simulink model "Copy_of_planar1R_2R"  (R2022b)
settings: Solver=VariableStepAuto  StartTime=0.0  StopTime=100  FixedStep=0.001  RelTol=1e-6
model workspace (MAT data in the model file):
  LC = Simulink.Signal
  LC.DataType = 'double'
  LC.Dimensions = 1
  LC.DimensionsMode = 'auto'
  LC.Complexity = 'real'
  LC.SampleTime = -1
  LC.SamplingMode = 'auto'
  LC.InitialValue = '1'
  fsA = Simulink.Signal
  fsA.DataType = 'double'
  fsA.Dimensions = 1
  fsA.DimensionsMode = 'auto'
  fsA.Complexity = 'real'
  fsA.SampleTime = -1
  fsA.SamplingMode = 'auto'
  fsA.InitialValue = '0.0'
  fsC = Simulink.Signal
  fsC.DataType = 'double'
  fsC.Dimensions = 1
  fsC.DimensionsMode = 'auto'
  fsC.Complexity = 'real'
  fsC.SampleTime = -1
  fsC.SamplingMode = 'auto'
  fsC.InitialValue = '0'
  fvA = Simulink.Signal
  fvA.DataType = 'double'
  fvA.Dimensions = 1
  fvA.DimensionsMode = 'auto'
  fvA.Complexity = 'real'
  fvA.SampleTime = -1
  fvA.SamplingMode = 'auto'
  fvA.InitialValue = '0.0'
  fvC = Simulink.Signal
  fvC.DataType = 'double'
  fvC.Dimensions = 1
  fvC.DimensionsMode = 'auto'
  fvC.Complexity = 'real'
  fvC.SampleTime = -1
  fvC.SamplingMode = 'auto'
  fvC.InitialValue = '0.0'
  g0 = Simulink.Signal
  g0.DataType = 'double'
  g0.Dimensions = 1
  g0.DimensionsMode = 'auto'
  g0.Complexity = 'real'
  g0.SampleTime = -1
  g0.SamplingMode = 'auto'
  g0.InitialValue = '9.8'
  iAxx = Simulink.Signal
  iAxx.DataType = 'double'
  iAxx.Dimensions = 1
  iAxx.DimensionsMode = 'auto'
  iAxx.Complexity = 'real'
  iAxx.SampleTime = -1
  iAxx.SamplingMode = 'auto'
  iAxx.InitialValue = '0.0'
  iCxx = Simulink.Signal
  iCxx.DataType = 'double'
  iCxx.Dimensions = 1
  iCxx.DimensionsMode = 'auto'
  iCxx.Complexity = 'real'
  iCxx.SampleTime = -1
  iCxx.SamplingMode = 'auto'
  iCxx.InitialValue = '0'
  lA = Simulink.Signal
  lA.DataType = 'double'
  lA.Dimensions = 1
  lA.DimensionsMode = 'auto'
  lA.Complexity = 'real'
  lA.SampleTime = -1
  lA.SamplingMode = 'auto'
  lA.InitialValue = '0.54'
  lC = Simulink.Signal
  lC.DataType = 'double'
  lC.Dimensions = 1
  lC.DimensionsMode = 'auto'
  lC.Complexity = 'real'
  lC.SampleTime = -1
  lC.SamplingMode = 'auto'
  lC.InitialValue = '1'
  mA = Simulink.Signal
  mA.DataType = 'double'
  mA.Dimensions = 1
  mA.DimensionsMode = 'auto'
  mA.Complexity = 'real'
  mA.SampleTime = -1
  mA.SamplingMode = 'auto'
  mA.InitialValue = '1'
  mC = Simulink.Signal
  mC.DataType = 'double'
  mC.Dimensions = 1
  mC.DimensionsMode = 'auto'
  mC.Complexity = 'real'
  mC.SampleTime = -1
  mC.SamplingMode = 'auto'
  mC.InitialValue = '1'
settings Model: Creator=giancarlo  LastModifiedBy=giancarlo

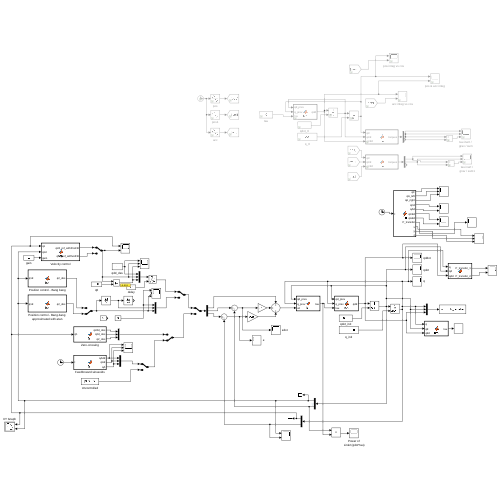
[thumbnail: Simulink's stored preview of the top-level diagram]
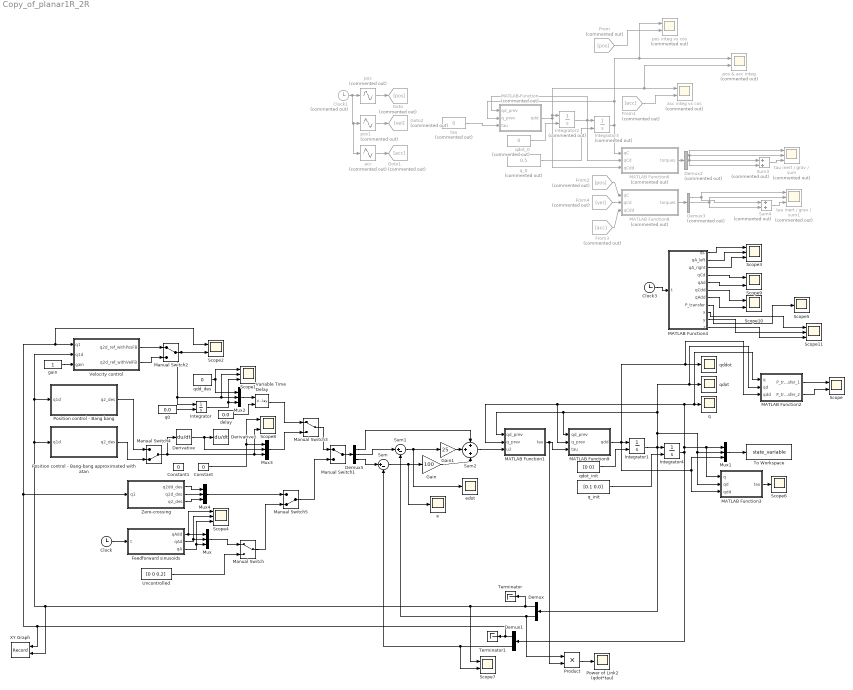
== system Copy_of_planar1R_2R ==
  Clock : Clock
  Clock1 : Clock  Commented=on
  Clock3 : Clock
  Constant : Constant  Value=0
  Constant1 : Constant  Value=0
  Demux : Demux  Outputs=2
  Demux1 : Demux  Outputs=2
  Demux2 : Demux  Commented=on  Outputs=[1 1 2 ]
  Demux3 : Demux  Commented=on  Outputs=[1 1 2 ]
  Demux5 : Demux  Outputs=3
  Derivative : Derivative
  Derivative1 : Derivative
  Feedforward sinusoids : MATLAB Function  TreatAsAtomicUnit=on
  From : From  Commented=on  GotoTag=pos
  From1 : From  Commented=on  GotoTag=acc
  From2 : From  Commented=on  GotoTag=pos
  From3 : From  Commented=on  GotoTag=acc
  From4 : From  Commented=on  GotoTag=vel
  Gain : Gain  Gain=100
  Gain1 : Gain  Gain=25
  Goto : Goto  Commented=on  GotoTag=pos
  Goto1 : Goto  Commented=on  GotoTag=acc
  Goto2 : Goto  Commented=on  GotoTag=vel
  Integrator : Integrator  InitialConditionSource=external  InitialCondition=0.3
  Integrator1 : Integrator  InitialConditionSource=external  InitialCondition=[0 0]
  Integrator2 : Integrator  Commented=on  InitialConditionSource=external  InitialCondition=[0 0]
  Integrator3 : Integrator  Commented=on  InitialConditionSource=external  InitialCondition=[0 0]
  Integrator4 : Integrator  InitialConditionSource=external  InitialCondition=[0 0]
  MATLAB Function : MATLAB Function  Commented=on  TreatAsAtomicUnit=on
  MATLAB Function1 : MATLAB Function  TreatAsAtomicUnit=on
  MATLAB Function2 : MATLAB Function  TreatAsAtomicUnit=on
  MATLAB Function3 : MATLAB Function  TreatAsAtomicUnit=on
  MATLAB Function4 : MATLAB Function  TreatAsAtomicUnit=on
  MATLAB Function6 : MATLAB Function  Commented=on  TreatAsAtomicUnit=on
  MATLAB Function8 : MATLAB Function  Commented=on  TreatAsAtomicUnit=on
  MATLAB Function9 : MATLAB Function  TreatAsAtomicUnit=on
  Manual Switch{,1..3} (4 alike) : ManualSwitch
  Manual Switch4 : ManualSwitch  CurrentSetting=0
  Manual Switch5 : ManualSwitch  CurrentSetting=0
  Mux{,1..4} (5 alike) : Mux  Inputs=3
  Position control - Bang bang : MATLAB Function  TreatAsAtomicUnit=on
  Position control - Bang-bang approximated with atan : MATLAB Function  TreatAsAtomicUnit=on
  Power of Link2 (qdot*tau) : Scope
  Product : Product
  Scope{,2,7,9..10} (5 alike) : Scope  NumInputPorts=2
  Scope{1,3..4,8,11} (5 alike) : Scope  NumInputPorts=3
  Scope5 : Scope
  Scope6 : Scope
  Sum : Sum  Inputs=|+-
  Sum1 : Sum  Inputs=|+-
  Sum2 : Sum  Inputs=+++
  Sum3 : Sum  Commented=on
  Sum4 : Sum  Commented=on
  Terminator : Terminator
  Terminator1 : Terminator
  To Workspace : ToWorkspace  VariableName=state_variable  SaveFormat=Timeseries  SampleTime=-1
  Uncontrolled : Constant  Value=[0 0 0.2]
  Variable Time Delay : VariableTransportDelay  MaximumDelay=10
  Velocity control : MATLAB Function  TreatAsAtomicUnit=on
  XY Graph : Record  FileSettingsInternal="{\"entries\":[{\"content\":{\"excelSettings\":{\"content\":{},\"type\":\"Streamout.ExcelSettings\"}},\"type\":\"Streamout.FileSettingStorage\",\"uuid\":\"17f3f7c0-a543-4966-915e-296ee2588332\"}],\"packageUris\":[\"http://schema.mathworks.com/mf0/streamout_blocks/R2020a\"],\"version\":\"1.0\"}"  Layout=[1 1]  SignalsInternal="{\"entries\":[{\"content\":{\"signals\":[{\"content\":{\"blockPath\":[\"Copy_of_planar1R_2R/XY Graph\"],\"channel\":[],\"dimensions\":[1],\"domain\":\"Copy_of_planar1R_2R/XY Graph\",\"lineColor\":\"#a2142f\",\"plots\":[1],\"port\":1,\"sid\":[\"\"],\"signalID\":42397,\"signalName\":\"Demux1:1\"},\"type\":\"RecordBlkView.Signal\",\"uuid\":\"0ab6503b-74ed-4c5b-b113-e67b91689d53\"},{\"content\":{\"blockPath\":[\"Copy_of_planar1R_2R/XY Graph\"],\"channel\":[],\"dimensions\":[1],\"domain\":\"Copy_of_planar1R_2R/XY Graph\",\"lineColor\":\"#139fff\",\"plots\":[1],\"port\":2,\"sid\":[\"\"],\"signalID\":42401,\"signalName\":\"Demux:1\"},\"type\":\"RecordBlkView.Signal\",\"uuid\":\"fae32842-6c35-404d-92af-908aeb941329\"}]},\"type\":\"RecordBlkView.InputSignals\",\"uuid\":\"726fd067-675c-490d-8cf4-42f1baed3ed2\"}],\"packageUris\":[\"http://schema.mathworks.com/mf0/streamout_blocks/R2020a\"],\"version\":\"1.0\"}"  VisualizationBindings="{\"xyplotplugin\":{\"info\":[{\"series\":[{\"bindingParametersList\":[{\"parameter\":\"X-Axis\",\"signalID\":42397,\"signalName\":\"Demux1:1\"},{\"parameter\":\"Y-Axis\",\"signalID\":42401,\"signalName\":\"Demux:1\"}],\"seriesID\":10957}],\"subplotID\":1}]}}"  CompatibilityTag=XY
  Zero-crossing : MATLAB Function  TreatAsAtomicUnit=on
  acc : Sin  Commented=on  TimeSource=Use external signal  Amplitude=-0.5*(2*pi*0.261145458563799)^2  Frequency=2*pi*0.261145458563799  Phase=pi/2  SampleTime=0
  acc integ vs cos : Scope  Commented=on  NumInputPorts=2
  delay : Constant  Value=0.0
  e : Scope
  edot : Scope
  gain : Constant
  pos : Sin  Commented=on  TimeSource=Use external signal  Amplitude=0.5  Frequency=2*pi*(0.261145458563799)  Phase=pi/2  SampleTime=0
  pos & acc integ : Scope  Commented=on  NumInputPorts=2
  pos integ vs cos : Scope  Commented=on  NumInputPorts=2
  pos1 : Sin  Commented=on  TimeSource=Use external signal  Amplitude=0.5*(2*pi*(0.261145458563799))  Frequency=2*pi*(0.261145458563799)  Phase=pi  SampleTime=0
  q : Scope
  q0 : Constant  Value=0.0
  q_0 : Constant  Commented=on  Value=0.5
  q_init : Constant  Value=[0.1 0.0]
  qdd_des : Constant  Value=0
  qddot : Scope
  qdot : Scope
  qdot_0 : Constant  Commented=on  Value=0
  qdot_init : Constant  Value=[0 0]
  tau : Constant  Commented=on  Value=0
  tau inert / grav / sum : Scope  Commented=on  NumInputPorts=3
  tau inert / grav / sum1 : Scope  Commented=on  NumInputPorts=3
  wires:
  qdot_0/1 -> Integrator2/2
  Integrator2/1 -> MATLAB Function6/2(qCd), MATLAB Function/1(qd_prev), Integrator3/1
  MATLAB Function/1(qdd) -> pos & acc integ/2, acc integ vs cos/1, Integrator2/1, MATLAB Function6/3(qCdd)
  q_0/1 -> Integrator3/2
  Integrator3/1 -> MATLAB Function6/1(qC), pos & acc integ/1, pos integ vs cos/1, MATLAB Function/2(q_prev)
  tau/1 -> MATLAB Function/3(tau)
  MATLAB Function6/1(torques) -> Demux2/1
  Demux2/1 -> Sum3/1, tau inert / grav / sum/1
  Demux2/2 -> tau inert / grav / sum/2, Sum3/2
  Sum3/1 -> tau inert / grav / sum/3
  From/1 -> pos integ vs cos/2
  From1/1 -> acc integ vs cos/2
  From2/1 -> MATLAB Function8/1(qC)
  From4/1 -> MATLAB Function8/2(qCd)
  Clock1/1 -> pos1/1, acc/1, pos/1
  pos/1 -> Goto/1
  acc/1 -> Goto1/1
  From3/1 -> MATLAB Function8/3(qCdd)
  pos1/1 -> Goto2/1
  Sum4/1 -> tau inert / grav / sum1/3
  MATLAB Function8/1(torques) -> Demux3/1
  Demux3/2 -> tau inert / grav / sum1/2, Sum4/2
  Demux3/1 -> Sum4/1, tau inert / grav / sum1/1
  Integrator4/1 -> Mux1/1, MATLAB Function3/1(q), MATLAB Function2/1(q), q/1, MATLAB Function1/2(q_prev), MATLAB Function9/2(q_prev), Demux1/1
  Demux/2 -> Sum1/2, Product/1
  Demux1/2 -> Scope7/2, Sum/2
  Gain1/1 -> Sum2/2
  q_init/1 -> Integrator4/2
  Sum/1 -> e/1, Gain/1
  Demux1/1 -> XY Graph/1, Scope2/1, Velocity control/1(q1), Zero-crossing/1(q1), Terminator1/1
  Sum1/1 -> Gain1/1, edot/1
  qdot_init/1 -> Integrator1/2
  MATLAB Function9/1(qdd) -> qddot/1, MATLAB Function2/3(qdd), Integrator1/1, Mux1/3, MATLAB Function3/3(qdd)
  Demux/1 -> Terminator/1, Scope7/1, XY Graph/2, Velocity control/2(q1d), Position control - Bang bang/1(q1d), Position control - Bang-bang approximated with atan/1(q1d)
  Gain/1 -> Sum2/3
  MATLAB Function1/1(tau) -> Product/2, MATLAB Function9/3(tau)
  Sum2/1 -> MATLAB Function1/3(u2)
  Clock/1 -> Feedforward sinusoids/1(t)
  Feedforward sinusoids/1(qAdd) -> Scope4/1, Mux/1
  Feedforward sinusoids/3(qA) -> Mux/3, Scope4/3
  Feedforward sinusoids/2(qAd) -> Scope4/2, Mux/2
  Manual Switch2/1 -> Scope2/2, Scope1/2, Mux2/2, Integrator/1
  q0/1 -> Integrator/2
  Uncontrolled/1 -> Manual Switch/2
  Mux/1 -> Manual Switch/1
  Demux5/1 -> Sum2/1
  Demux5/2 -> Sum1/1
  Demux5/3 -> Sum/1
  Mux1/1 -> To Workspace/1
  Integrator1/1 -> qdot/1, MATLAB Function2/2(qd), MATLAB Function9/1(qd_prev), MATLAB Function1/1(qd_prev), MATLAB Function3/2(qd), Mux1/2, Demux/1, Integrator4/1
  MATLAB Function3/1(tau) -> Scope6/1
  Manual Switch1/1 -> Demux5/1
  Mux2/1 -> Variable Time Delay/1
  Integrator/1 -> Mux2/3, Scope1/3
  qdd_des/1 -> Mux2/1, Scope1/1
  delay/1 -> Variable Time Delay/2
  gain/1 -> Velocity control/3(gain)
  Velocity control/1(q2d_ref_withPosFB) -> Manual Switch2/1
  Velocity control/2(q2d_ref_withVelFB) -> Manual Switch2/2
  Mux3/1 -> Manual Switch3/2
  Variable Time Delay/1 -> Manual Switch3/1
  Manual Switch3/1 -> Manual Switch1/1
  Product/1 -> Power of Link2 (qdot*tau)/1
  Constant/1 -> Scope8/1, Mux3/1
  Position control - Bang-bang approximated with atan/1(q2_des) -> Manual Switch4/2
  Position control - Bang bang/1(q2_des) -> Manual Switch4/1
  Manual Switch4/1 -> Scope8/3, Mux3/3, Derivative/1
  Derivative/1 -> Mux3/2, Derivative1/1
  Zero-crossing/1(q2dd_des) -> Mux4/1
  Zero-crossing/2(q2d_des) -> Mux4/2
  Zero-crossing/3(q2_des) -> Mux4/3
  Manual Switch/1 -> Manual Switch5/2
  Manual Switch5/1 -> Manual Switch1/2
  Mux4/1 -> Manual Switch5/1
  MATLAB Function2/2(P_transfer_2) -> Scope/2
  MATLAB Function2/1(P_transfer_1) -> Scope/1
  Clock3/1 -> MATLAB Function4/1(t)
  MATLAB Function4/8(P_transfer) -> Scope5/1
  MATLAB Function4/1(qC) -> Scope3/1
  MATLAB Function4/2(qA_left) -> Scope3/2
  MATLAB Function4/4(qCd) -> Scope9/1
  MATLAB Function4/5(qAd) -> Scope9/2
  MATLAB Function4/6(qCdd) -> Scope10/1
  MATLAB Function4/7(qAdd) -> Scope10/2
  MATLAB Function4/3(qA_right) -> Scope3/3
  MATLAB Function4/9(x) -> Scope11/1
  MATLAB Function4/10(y) -> Scope11/2
  MATLAB Function4/11(z) -> Scope11/3

== matlab function Copy_of_planar1R_2R/Position control - Bang bang ==
  settings: updateMethod=DISCRETE  sampleTime=0.0001
  data: q1d input; q2_des output
function q2_des = fcn(q1d)

alpha = -0.2;
q2_des = alpha*sign(q1d);

end

== matlab function Copy_of_planar1R_2R/Position control - Bang-bang approximated with atan ==
  settings: updateMethod=DISCRETE  sampleTime=0.0001
  data: q2_des output; q1d input
function q2_des = fcn(q1d)

alpha = -2;
q2_des = alpha*atan(q1d);

end

== matlab function Copy_of_planar1R_2R/MATLAB Function6 ==
  settings: updateMethod=DISCRETE  sampleTime=0.001
  data: qC input; torques output; qCd input; qCdd input; mC data_store_memory; lC data_store_memory; iCxx data_store_memory; fvC data_store_memory; fsC data_store_memory; g0 data_store_memory
function torques = fcn(qC, qCd, qCdd)
global mC lC iCxx fvC fsC g0

tau_inert = qCdd*(mC*lC^2 + iCxx);
tau_grav = g0*lC*mC*sin(qC);
tau_visc_fric = fvC*qCd;
tau_stat_fric = fsC*sign(qCd);

torques = [tau_inert; tau_grav; tau_visc_fric; tau_stat_fric];

end

== matlab function Copy_of_planar1R_2R/MATLAB Function8 ==
  settings: updateMethod=DISCRETE  sampleTime=0.001
  data: qC input; torques output; qCd input; qCdd input; mC data_store_memory; lC data_store_memory; iCxx data_store_memory; fvC data_store_memory; fsC data_store_memory; g0 data_store_memory
function torques = fcn(qC, qCd, qCdd)
global mC lC iCxx fvC fsC g0

tau_inert = qCdd*(mC*lC^2 + iCxx);
tau_grav = g0*lC*mC*sin(qC);
tau_visc_fric = fvC*qCd;
tau_stat_fric = fsC*sign(qCd);

torques = [tau_inert; tau_grav; tau_visc_fric; tau_stat_fric];

end

== matlab function Copy_of_planar1R_2R/Feedforward sinusoids ==
  settings: updateMethod=DISCRETE  sampleTime=0.0001
  data: qAdd output; qAd output; qA output; t input
function [qAdd, qAd, qA] = fcn(t)

period = 3.8907;
% period = 4;
f = 1/period;
phi = 0;
A = 0.2;

qA = A*cos(2*pi*f*t + phi);
qAd = -(A*2*pi*f)*sin(2*pi*f*t + phi);
qAdd = -A*(2*pi*f)^2*cos(2*pi*f*t + phi);

% omega = 2*pi*f;
% decay_rate = 0.005;
% 
% qA = A * exp(-decay_rate*t) * cos(omega*t + phi);
% qAd = -A * exp(-decay_rate*t) * (decay_rate * cos(phi + omega*t) + omega * sin(phi + omega * t));
% qAdd = A * exp(-decay_rate*t) * (decay_rate^2 * cos(phi + omega*t) - omega^2  * cos(phi + omega*t) + 2*decay_rate*omega*sin(phi + omega*t));

end

== matlab function Copy_of_planar1R_2R/MATLAB Function9 ==
  settings: updateMethod=DISCRETE  sampleTime=0.0001
  data: qd_prev input; q_prev input; tau input; qdd output; mC data_store_memory; lC data_store_memory; iCxx data_store_memory; fsC data_store_memory; fvC data_store_memory; g0 data_store_memory; mA data_store_memory; LC data_store_memory; lA data_store_memory; iAxx data_store_memory; fvA data_store_memory; fsA data_store_memory
function qdd = fcn(qd_prev, q_prev, tau)

global mC lC iCxx fvC fsC g0 LC lA mA iAxx fvA fsA

qC = q_prev(1);
qA = q_prev(2);
qCd = qd_prev(1);
qAd = qd_prev(2);

qdd = [0;0];

B = [mA*LC^2 + 2*mA*cos(qA)*LC*lA + mA*lA^2 + mC*lC^2 + iAxx + iCxx, mA*lA^2 + LC*mA*cos(qA)*lA + iAxx;
                                 mA*lA^2 + LC*mA*cos(qA)*lA + iAxx,                    mA*lA^2 + iAxx];

n = [- LC*lA*mA*sin(qA)*qAd^2 - 2*LC*lA*mA*qCd*sin(qA)*qAd + fvC*qCd + fsC*sign(qCd) + g0*lA*mA*sin(qA + qC) + LC*g0*mA*sin(qC) + g0*lC*mC*sin(qC);
                                                                        LC*lA*mA*sin(qA)*qCd^2 + fvA*qAd + fsA*sign(qAd) + g0*lA*mA*sin(qA + qC)];

% B = [mA*LC^2 + 2*mA*cos(qA)*LC*lA + mA*lA^2 + mC*lC^2 + iAxx + iCxx, 0;
%                                  0,                    mA*lA^2 + iAxx];
% 
% n = [- LC*lA*mA*sin(qA)*qAd^2 - 2*LC*lA*mA*qCd*sin(qA)*qAd + fvC*qCd + fsC*sign(qCd) + g0*lA*mA*sin(qA + qC) + LC*g0*mA*sin(qC) + g0*lC*mC*sin(qC);
%                                                                         LC*lA*mA*sin(qA)*qCd^2 + fvA*qAd + fsA*sign(qAd) + g0*lA*mA*sin(qA + qC)];

% Direct dynamics
G = [0;
     1];

qdd = inv(B)*(G*tau-n);

end

== matlab function Copy_of_planar1R_2R/Zero-crossing ==
  settings: updateMethod=DISCRETE  sampleTime=0.0001
  data: q2dd_des output; q2d_des output; q2_des output; q1 input
function [q2dd_des, q2d_des, q2_des] = fcn(q1)

alpha = 0.3;

q2dd_des = 0;
q2d_des = 0;
q2_des = alpha*sign(q1);

end

== matlab function Copy_of_planar1R_2R/MATLAB Function2 ==
  settings: updateMethod=DISCRETE  sampleTime=0.0001
  data: P_transfer_1 output; q input; qd input; qdd input; P_transfer_2 output; mC data_store_memory; lC data_store_memory; iCxx data_store_memory; fsC data_store_memory; fvC data_store_memory; g0 data_store_memory; mA data_store_memory; LC data_store_memory; lA data_store_memory; iAxx data_store_memory; fvA data_store_memory; fsA data_store_memory
function [P_transfer_1, P_transfer_2] = fcn(q, qd, qdd)

global mC lC iCxx fvC fsC g0 LC lA mA iAxx fvA fsA

qC = q(1);
qA = q(2);
qCd = qd(1);
qAd = qd(2);
qCdd = qdd(1);
qAdd = qdd(2);


P_transfer = mA*lC*lA*(qCdd*qAd*cos(qC-qA) + qCd*qAdd*cos(qC-qA) - qCd*qAd*sin(qC-qA)*(qCd-qAd));

P_transfer_1 = mA*lC*lA*(qCd*qAdd*cos(qC-qA));
P_transfer_2 = mA*lC*lA*(qAd*qCdd*cos(qC-qA));

end

== matlab function Copy_of_planar1R_2R/MATLAB Function4 ==
  settings: updateMethod=DISCRETE  sampleTime=0.0001
  data: qC output; qA_left output; qA_right output; qCd output; qAd output; qCdd output; qAdd output; P_transfer output; t input; mC data_store_memory; lC data_store_memory; iCxx data_store_memory; fsC data_store_memory; fvC data_store_memory; g0 data_store_memory; mA data_store_memory; LC data_store_memory; lA data_store_memory; iAxx data_store_memory; fvA data_store_memory; fsA data_store_memory; x output; y output; z output
function [qC, qA_left, qA_right, qCd, qAd, qCdd, qAdd, P_transfer, x, y, z] = fcn(t)

global mC lC iCxx fvC fsC g0 LC lA mA iAxx fvA fsA

period = 3.8907;
% period = 4;
f = 1/period;
omega = 2*pi*f;
phi1 = 0;
phi2 = -90*pi/180;
A1 = 0.1;
A2 = 0.1;

qC = A1*cos(omega*t + phi1);
qCd = -(A1*omega)*sin(omega*t + phi1);
qCdd = -A1*omega^2*cos(omega*t + phi1);

shift = -0*pi/180;
% shift = -0;
qA_left = A2*cos(omega*t + phi2) + shift;
qA_right= A2*cos(omega*t + phi2) - shift;
qAd = -(A2*omega)*sin(omega*t + phi2);
qAdd = -A2*omega^2*cos(omega*t + phi2);

% P_transfer = mA*lC*lA*qAdd*cos(qC-qA_left)*qCd + mA*lC*lA*qAdd*cos(qC-qA_right)*qCd;

P_transfer = mA*lC*lA*qAdd*cos(qC-qA_left)*qCd;
x = 1/2*sin(2*omega*t + phi2);
y = 1/2*sin(phi2);
z = A1*cos(omega*t) - A2*cos(omega*t + phi2);

end

== matlab function Copy_of_planar1R_2R/MATLAB Function1 ==
  settings: updateMethod=DISCRETE  sampleTime=0.0001
  data: qd_prev input; q_prev input; u2 input; tau output; mC data_store_memory; lC data_store_memory; iCxx data_store_memory; fsC data_store_memory; fvC data_store_memory; g0 data_store_memory; mA data_store_memory; LC data_store_memory; lA data_store_memory; iAxx data_store_memory; fvA data_store_memory; fsA data_store_memory
function tau = fcn(qd_prev, q_prev, u2)
global mC lC iCxx fvC fsC g0 LC lA mA iAxx fvA fsA


qC = q_prev(1);
qA = q_prev(2);
qCd = qd_prev(1);
qAd = qd_prev(2);

B = [mA*LC^2 + 2*mA*cos(qA)*LC*lA + mA*lA^2 + mC*lC^2 + iAxx + iCxx, mA*lA^2 + LC*mA*cos(qA)*lA + iAxx;
                                 mA*lA^2 + LC*mA*cos(qA)*lA + iAxx,                    mA*lA^2 + iAxx];

n = [- LC*lA*mA*sin(qA)*qAd^2 - 2*LC*lA*mA*qCd*sin(qA)*qAd + fvC*qCd + fsC*sign(qCd) + g0*lA*mA*sin(qA + qC) + LC*g0*mA*sin(qC) + g0*lC*mC*sin(qC);
                                                                        LC*lA*mA*sin(qA)*qCd^2 + fvA*qAd + fsA*sign(qAd) + g0*lA*mA*sin(qA + qC)];

% B = [mA*LC^2 + 2*mA*cos(qA)*LC*lA + mA*lA^2 + mC*lC^2 + iAxx + iCxx, 0;
%                                  0,                    mA*lA^2 + iAxx];

% n = [- LC*lA*mA*sin(qA)*qAd^2 - 2*LC*lA*mA*qCd*sin(qA)*qAd + fvC*qCd + fsC*sign(qCd) + g0*lA*mA*sin(qA + qC) + LC*g0*mA*sin(qC) + g0*lC*mC*sin(qC);
%                                                                         LC*lA*mA*sin(qA)*qCd^2 + fvA*qAd + fsA*sign(qAd) + g0*lA*mA*sin(qA + qC)];

% Collocated PFBL
b11 = B(1,1);
b12 = B(1,2);
b21 = B(2,1);
b22 = B(2,2);
n1 = n(1);
n2 = n(2);

tau = (b22 - b21*inv(b11)*b12)*u2 + n2 - b21*inv(b11)*n1;

end

== matlab function Copy_of_planar1R_2R/MATLAB Function ==
  settings: updateMethod=DISCRETE  sampleTime=0.001
  data: qd_prev input; q_prev input; tau input; qdd output; mC data_store_memory; lC data_store_memory; iCxx data_store_memory; fsC data_store_memory; fvC data_store_memory; g0 data_store_memory
function qdd = fcn(qd_prev, q_prev, tau)

global mC lC iCxx fvC fsC g0
qC = q_prev;
qCd = qd_prev;

B = mC*lC^2 + iCxx;
n = fvC*qCd + fsC*sign(qCd) + g0*lC*mC*sin(qC);

% Direct dynamics
qdd = (B)\(tau-n);

end

== matlab function Copy_of_planar1R_2R/Velocity control ==
  settings: updateMethod=DISCRETE  sampleTime=0.0001
  data: q1 input; q1d input; q2d_ref_withPosFB output; gain input; q2d_ref_withVelFB output
function [q2d_ref_withPosFB, q2d_ref_withVelFB] = fcn(q1, q1d, gain)

maxVel = 0.57;
q2d_ref_withPosFB = maxVel*tanh(gain*q1);

q2d_ref_withVelFB = gain*q1d;

end

== matlab function Copy_of_planar1R_2R/MATLAB Function3 ==
  settings: updateMethod=DISCRETE  sampleTime=0.0001
  data: q input; qd input; qdd input; tau output; mC data_store_memory; lC data_store_memory; iCxx data_store_memory; fsC data_store_memory; fvC data_store_memory; g0 data_store_memory; mA data_store_memory; LC data_store_memory; lA data_store_memory; iAxx data_store_memory; fvA data_store_memory; fsA data_store_memory
function tau = fcn(q, qd, qdd)

global mC lC iCxx fvC fsC g0 LC lA mA iAxx fvA fsA

qC = q(1);
qA = q(2);
qCd = qd(1);
qAd = qd(2);
qCdd = qdd(1);
qAdd = qdd(2);

B = [mA*LC^2 + 2*mA*cos(qA)*LC*lA + mA*lA^2 + mC*lC^2 + iAxx + iCxx, mA*lA^2 + LC*mA*cos(qA)*lA + iAxx;
                                 mA*lA^2 + LC*mA*cos(qA)*lA + iAxx,                    mA*lA^2 + iAxx];

n = [- LC*lA*mA*sin(qA)*qAd^2 - 2*LC*lA*mA*qCd*sin(qA)*qAd + fvC*qCd + fsC*sign(qCd) + g0*lA*mA*sin(qA + qC) + LC*g0*mA*sin(qC) + g0*lC*mC*sin(qC);
                                                                        LC*lA*mA*sin(qA)*qCd^2 + fvA*qAd + fsA*sign(qAd) + g0*lA*mA*sin(qA + qC)];

tau = B*qdd + n;

end
